simulink library "Pressure_Drop_Fix"  (Simulink 8.2)
settings: Solver=ode45  StartTime=0.0  StopTime=10.0  RelTol=1e-3
undefined symbols (not defined in the file): con, DPConstant, DPLinear, DPQuadratic, lin, Pressure, qua
libraries: simulink x2, carnot x1
settings Model: Creator=drhf  LastModifiedBy=drhf

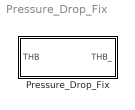
== system Pressure_Drop_Fix ==
  Pressure_Drop_Fix : Subsystem  mask(fixed pressure drop){con=con, lin=lin, qua=qua}
      mask prompts: con "c : constant (static) pressure drop in Pa"; lin "l : linear pressure drop Pa/(kg/s)"; qua "q : quadratic pressure drop Pa/(kg/s)²"
      mask help:
      | Constant parameters for pressure drop in a flow.
      | dp = c + l*mdot + q*mdot²
      | Calculation is done for ID > 10000 (dp = f(l, q), c is neglected) and ID > 20000 (dp = f(c,l,q)).
      | Applied directly to the THB bus.
      mask Help: web(fullfile(path_carnot('help'),'Pressure_Drop_Fix.html'),'-helpbrowser')

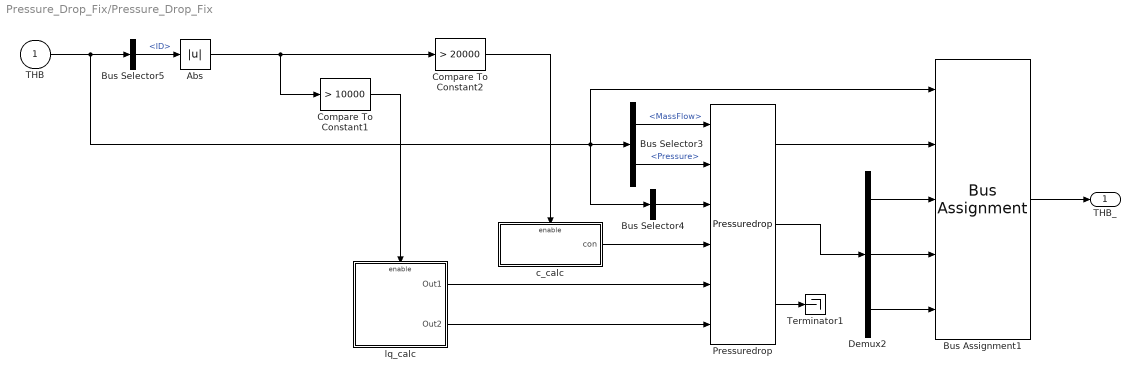
== system Pressure_Drop_Fix/Pressure_Drop_Fix ==
  THB : Inport
  Abs : Abs
  Bus Assignment1 : BusAssignment  AssignedSignals=Pressure,DPConstant,DPLinear,DPQuadratic
  Bus Selector3 : BusSelector  OutputSignals=MassFlow,Pressure
  Bus Selector4 : BusSelector  OutputSignals=DPConstant,DPLinear,DPQuadratic  OutputAsBus=on
  Bus Selector5 : BusSelector  OutputSignals=ID
  Compare To Constant1 : simulink/Logic and Bit Operations/Compare To Constant  relop=>  const=10000  OutDataTypeStr=boolean
  Compare To Constant2 : simulink/Logic and Bit Operations/Compare To Constant  relop=>  const=20000  OutDataTypeStr=boolean
  Demux2 : Demux  Outputs=3
  Pressuredrop : carnot/Basic/Pressure_Drop/Pressuredrop
  Terminator1 : Terminator
  c_calc : Subsystem
  lq_calc : Subsystem
  THB_ : Outport
  wires:
  Compare To Constant1/1 -> lq_calc/Enable
  lq_calc/2(Out2) -> Pressuredrop/6
  lq_calc/1(Out1) -> Pressuredrop/5
  Demux2/3 -> Bus Assignment1/5
  Demux2/2 -> Bus Assignment1/4
  Demux2/1 -> Bus Assignment1/3
  Bus Assignment1/1 -> THB_/1
  Pressuredrop/1 -> Bus Assignment1/2
  THB/1 -> Bus Assignment1/1, Bus Selector4/1, Bus Selector3/1, Bus Selector5/1
  Abs/1 -> Compare To Constant2/1, Compare To Constant1/1
  Bus Selector4/1 -> Pressuredrop/3
  Bus Selector3/1 -> Pressuredrop/1  "<MassFlow>"
  Bus Selector3/2 -> Pressuredrop/2  "<Pressure>"
  Bus Selector5/1 -> Abs/1  "<ID>"
  Compare To Constant2/1 -> c_calc/Enable
  c_calc/1(con) -> Pressuredrop/4
  Pressuredrop/2 -> Demux2/1
  Pressuredrop/3 -> Terminator1/1

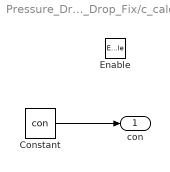
== system Pressure_Drop_Fix/Pressure_Drop_Fix/c_calc ==
  Enable : EnablePort
  Constant : Constant  Value=con
  con : Outport  InitialOutput=con
  wires:
  Constant/1 -> con/1

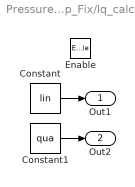
== system Pressure_Drop_Fix/Pressure_Drop_Fix/lq_calc ==
  Enable : EnablePort
  Constant : Constant  Value=lin
  Constant1 : Constant  Value=qua
  Out1 : Outport  InitialOutput=lin
  Out2 : Outport  Port=2  InitialOutput=qua
  wires:
  Constant1/1 -> Out2/1
  Constant/1 -> Out1/1
